simulink model "verify_EBcreator_mdl"  (R2018b)
settings: Solver=VariableStepDiscrete  StartTime=0.0  StopTime=10.0  MaxStep=0.1  RelTol=1e-3  EnableMultiTasking=on
libraries: carnot x1
settings Model: Creator=drhf  LastModifiedBy=drhf
settings DataIOCC: LimitDataPoints=on  SaveFormat=Array
settings OptimizationCC: ExpressionDepthLimit=2147483647  LifeSpan=inf
settings DebuggingCC: UnderspecifiedInitializationDetection=Classic  MergeDetectMultiDrivingBlocksExec=none  SolverPrmCheckMsg=warning  StateNameClashWarn=warning  SFUnexpectedBacktrackingDiag=warning  SFNoUnconditionalDefaultTransitionDiag=warning  SFExecutionAtInitializationDiag=none
settings HardwareCC: ProdBitPerPointer=32  ProdBitPerSizeT=32  ProdBitPerPtrDiffT=32  ProdLargestAtomicFloat=None  ProdIntDivRoundTo=Undefined  ProdEndianess=Unspecified  ProdWordSize=32  ProdHWDeviceType=32-bit Generic
settings ModelReferenceCC: PropagateSignalLabelsOutOfModel=off
settings SFSimCC: SimUseLocalCustomCode=off
settings RTWCC: RTWUseLocalCustomCode=off
settings CodeAppCC: StateflowObjectComments=on
settings GRTTargetCC: TargetLangStandard=C89/C90 (ANSI)  GeneratePreprocessorConditionals=Disable all  CombineOutputUpdateFcns=off  GRTInterface=on
settings ConfigComp: CovMetricSettings=dw  CovHtmlReporting=on  CovSaveCumulativeToWorkspaceVar=on  CovSaveSingleToWorkspaceVar=on  CovExternalEMLEnable=off

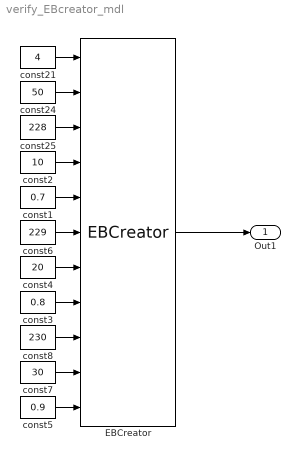
== system verify_EBcreator_mdl ==
  EBCreator : carnot/Basic/Electric/EBCreator  Inport_ID=on  Inport_f=on  Inport_v1=on  Inport_p1=on  Inport_pf1=on  Inport_v2=on  Inport_p2=on  Inport_pf2=on  Inport_v3=on  Inport_p3=on  Inport_pf3=on  ID=4  f=50  v1=230  p1=0  pf1=1  v2=230  p2=0  pf2=1  v3=230  p3=0  pf3=1  Annotation_ID=off  Annotation_f=off  Annotation_v1=off  Annotation_p1=off  Annotation_pf1=off  Annotation_v2=off  Annotation_p2=off  Annotation_pf2=off  Annotation_v3=off  Annotation_p3=off  Annotation_pf3=on
  const1 : Constant  Value=0.7
  const2 : Constant  Value=10
  const21 : Constant  Value=4
  const24 : Constant  Value=50
  const25 : Constant  Value=228
  const3 : Constant  Value=0.8
  const4 : Constant  Value=20
  const5 : Constant  Value=0.9
  const6 : Constant  Value=229
  const7 : Constant  Value=30
  const8 : Constant  Value=230
  Out1 : Outport
  wires:
  EBCreator/1 -> Out1/1
  const21/1 -> EBCreator/1
  const24/1 -> EBCreator/2
  const25/1 -> EBCreator/3
  const1/1 -> EBCreator/5
  const2/1 -> EBCreator/4
  const4/1 -> EBCreator/7
  const6/1 -> EBCreator/6
  const3/1 -> EBCreator/8
  const5/1 -> EBCreator/11
  const8/1 -> EBCreator/9
  const7/1 -> EBCreator/10
